simulink model "nid_cvst_point_cloud"  (Simulink 10.0)
settings: Solver=FixedStepDiscrete  StartTime=0.0  StopTime=inf  RelTol=1e-3  EnableMultiTasking=on
libraries: nid_lib x3, vipsnks x1
settings Model: Creator=tchikama  LastModifiedBy=bhisma
settings DataIOCC: LimitDataPoints=on  SignalLoggingSaveFormat=ModelDataLogs  SaveOutput=off  SaveTime=off
settings OptimizationCC: ExpressionDepthLimit=2147483647  SimCompilerOptimization=on
settings DebuggingCC: SolverPrmCheckMsg=warning  InheritedTsInSrcMsg=none  FcnCallInpInsideContextMsg=warning  StateNameClashWarn=warning
settings HardwareCC: ProdIntDivRoundTo=Zero  ProdEndianess=LittleEndian  ProdHWDeviceType=Generic->32-bit x86 compatible
settings RTWCC: RTWCompilerOptimization=on
settings CodeAppCC: MaxIdLength=95
settings GRTTargetCC: GeneratePreprocessorConditionals=Disable all
settings ConfigComp: CovExternalEMLEnable=off

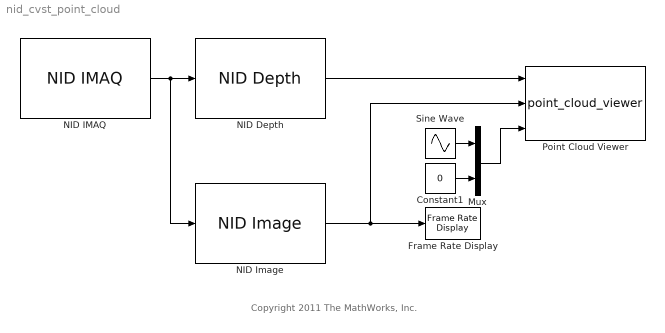
== system nid_cvst_point_cloud ==
  note: Copyright 2011 The MathWorks, Inc.
  Constant1 : Constant  Value=0
  Frame Rate Display : vipsnks/Frame Rate Display  UpdateRate=10
      settings: SourceProductName=Computer Vision Toolbox  SourceProductBaseCode=VP
  Mux : Mux  Inputs=2
  NID Depth : nid_lib/NID Depth  depthOutput=XYZ  conv_XYZ_RW=on  viewer=off
  NID IMAQ : nid_lib/NID IMAQ  imaq_depth=on  imaq_motion=off  imaq_image=on  view_point=on  imaq_skeleton=off  imaq_ir=off  mirror_image=off  imaq_sample_time=1/30  res_fps=VGA (640x480): 30 FPS  angle=0  angle_read=off  near_mode=off
  NID Image : nid_lib/NID Image  imageOutput=RGB
  Point Cloud Viewer : M-S-Function  FunctionName=point_cloud_viewer  Parameters=view  mask{view=off}
      mask prompts: view "Enable view signal"
      mask Display:
      | disp('Point Cloud \nViewer')
      | 
      | port_label('input', 1, 'XYZ')
      | port_label('input', 2, 'Image')
      | port_label('input', 3, 'View')
  Sine Wave : Sin  Amplitude=90  Frequency=0.2  Samples=720
  wires:
  NID IMAQ/1 -> NID Depth/1, NID Image/1
  NID Depth/1 -> Point Cloud Viewer/1
  NID Image/1 -> Point Cloud Viewer/2, Frame Rate Display/1
  Mux/1 -> Point Cloud Viewer/3
  Sine Wave/1 -> Mux/1
  Constant1/1 -> Mux/2
